simulink model "Simulations_section74"  (R2023a)
settings: Solver=ode15s  StartTime=0.0  StopTime=time_end  FixedStep=Ts  MaxStep=1e-3  RelTol=1e-3
values from neighbouring files (symbols this model uses):
  Akmax = CorrM.a    [Section74.m]
  Akmin = Corrm.a    [Section74.m]
  Bkmax = CorrM.b    [Section74.m]
  Bkmin = Corrm.b    [Section74.m]
  Ckmax = CorrM.c    [Section74.m]
  Ckmin = Corrm.c    [Section74.m]
  rhomax = 0.99    [Section74.m]
  rhomin = 0.01    [Section74.m]
  scenario = input('Which scenario would you like to run: 1 or 2 ? Answer = ')    [Section74.m]
undefined symbols (not defined in the file or in its folder): sigbuilder_block
libraries: cstblocks x6
settings Model: ExtModeTrigDuration=100000  Creator=senameo  LastModifiedBy=senameo
settings DataIOCC: SaveFormat=Array  SignalLoggingSaveFormat=ModelDataLogs  ReturnWorkspaceOutputs=off
settings OptimizationCC: BlockReduction=off  BooleanDataType=off  InitFltsAndDblsToZero=on  LifeSpan=inf
settings DebuggingCC: SaveWithParameterizedLinksMsg=none  UnderspecifiedInitializationDetection=Classic  MergeDetectMultiDrivingBlocksExec=none  SignalResolutionControl=TryResolveAllWithWarning  MultiTaskDSMMsg=warning  MultiTaskCondExecSysMsg=none  FcnCallInpInsideContextMsg=warning  UnconnectedInputMsg=warning  UnconnectedOutputMsg=warning  UnconnectedLineMsg=warning  SFUnexpectedBacktrackingDiag=warning  SFNoUnconditionalDefaultTransitionDiag=warning  SFExecutionAtInitializationDiag=none  ArithmeticOperatorsInVariantConditions=warning
settings HardwareCC: ProdBitPerPointer=32  ProdBitPerSizeT=32  ProdBitPerPtrDiffT=32  ProdLargestAtomicFloat=None  ProdIntDivRoundTo=Undefined  ProdEndianess=Unspecified  ProdWordSize=32  ProdHWDeviceType=32-bit Generic  TargetUnknown=on
settings ModelReferenceCC: EnableRefExpFcnMdlSchedulingChecks=on  PropagateSignalLabelsOutOfModel=off
settings RTWCC: SystemTargetFile=win_watc.tlc  TemplateMakefile=win_watc.tmf  DLArmComputeVersion=19.05
settings CodeAppCC: StateflowObjectComments=on
settings STFCustomTargetCC: TargetFcnLib=ansi_tfl_tmw.mat  TargetLangStandard=C89/C90 (ANSI)  ModelReferenceCompliant=off  ConcurrentExecutionCompliant=off  MATLABClassNameForMDSCustomization=Simulink.SoftwareTarget.TargetSpecificTriggerConfigurationBase  UseToolchainInfoCompliant=off  SystemTargetFile=win_watc.tlc
settings ConfigComp: CovMetricSettings=dw  CovSaveCumulativeToWorkspaceVar=on  CovSaveSingleToWorkspaceVar=on

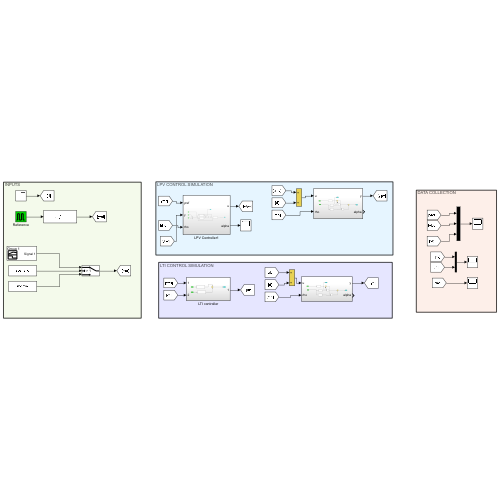
[thumbnail: Simulink's stored preview of the top-level diagram]
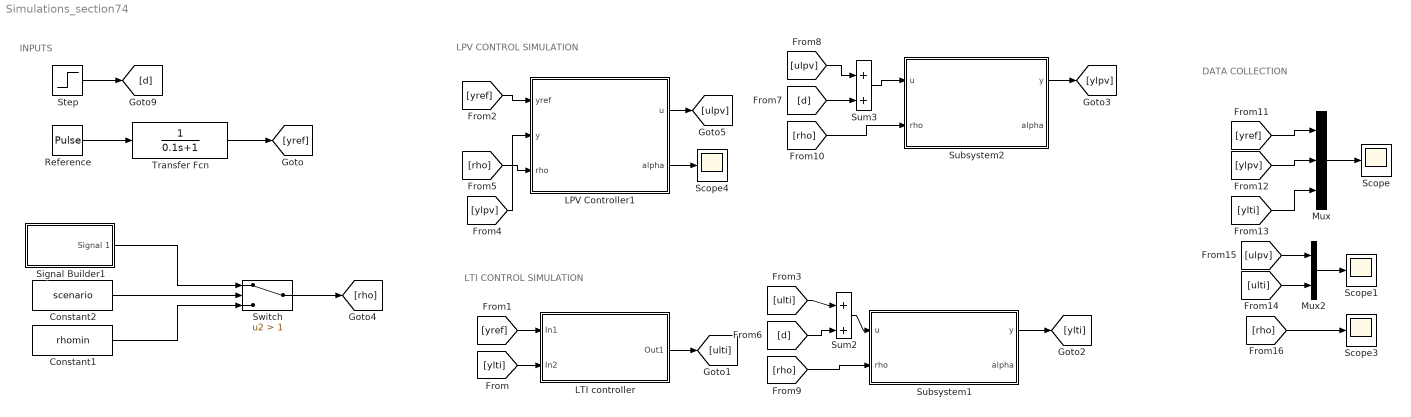
== system Simulations_section74 ==
  note: DATA COLLECTION
  note: LPV CONTROL SIMULATION
  note: LTI CONTROL SIMULATION
  note: INPUTS
  Constant1 : Constant  Value=rhomin
  Constant2 : Constant  Value=scenario
  LPV Controller1 : Subsystem
  LTI controller : Subsystem
  Mux : Mux  Inputs=3
  Mux2 : Mux  Inputs=2
  Reference : DiscretePulseGenerator  PulseType=Time based  Period=30  PulseWidth=50  PhaseDelay=1
  Scope{,1,3..4} (4 alike) : Scope
  Signal Builder1 : Subsystem  Tag=STV Subsys  LoadFcn=sigbuilder_block('load');  StartFcn=sigbuilder_block('start');  StopFcn=sigbuilder_block('stop');  ClipboardFcn=sigbuilder_block('clipboard');  mask(Sigbuilder block){tuvar=[0:10]}
      mask help: Simulink:masks:SigbuilderBlock_MD
      mask init:
      | if ~strcmp(get_param(bdroot(gcbh),'SimulationStatus'),'stopped') tuvar = sigbuilder_block('maskInit'); end
      settings: CopyFcn=sigbuilder_block('copy');  DeleteFcn=sigbuilder_block('delete');  ModelCloseFcn=sigbuilder_block('modelClose');  PreSaveFcn=sigbuilder_block('preSave');  PauseFcn=sigbuilder_block('pause');  ContinueFcn=sigbuilder_block('continue');  NameChangeFcn=sigbuilder_block('namechange');  OpenFcn=sigbuilder_block('open',[597 9 550.2 191.1 ]);  CloseFcn=sigbuilder_block('close');
      mask Display: plot(0, 0, 100, 100,[2, 2, 32, 32, 2], [68, 8, 8, 68, 68],[32, 2], [38, 38], [32, 19, 2],[53, 60, 44], [32, 17, 17, 2],[16, 16, 31, 31]);txt = getActiveGroup(gcbh);text(2, 100, txt,'verticalAlignment', 'top');
  Step : Step  Time=20  After=0.1  SampleTime=0
  Subsystem1 : Subsystem
  Subsystem2 : Subsystem
  Sum2 : Sum  Inputs=+|+  InputSameDT=on  SaturateOnIntegerOverflow=on  OutDataTypeStr=Inherit: Same as first input
  Sum3 : Sum  Inputs=+|+  InputSameDT=on  SaturateOnIntegerOverflow=on  OutDataTypeStr=Inherit: Same as first input
  Switch : Switch  Criteria=u2 > Threshold  Threshold=1  SaturateOnIntegerOverflow=off  InputSameDT=off
  Transfer Fcn : TransferFcn  Denominator=[0.1 1]
  wires:
  Sum2/1 -> Subsystem1/1(u)
  Mux2/1 -> Scope1/1
  Transfer Fcn/1 -> [yref]
  Reference/1 -> Transfer Fcn/1
  Mux/1 -> Scope/1
  [yref] -> LTI controller/1(In1)
  [ylti] -> LTI controller/2(In2)
  LTI controller/1(Out1) -> [ulti]
  [ulti] -> Sum2/1
  [d] -> Sum2/2
  [rho] -> Subsystem1/2(rho)
  [yref] -> Mux/1
  Subsystem1/1(y) -> [ylti]
  [ylpv] -> Mux/2
  [ulti] -> Mux2/2
  [ulpv] -> Mux2/1
  Constant2/1 -> Switch/2
  Switch/1 -> [rho]
  Step/1 -> [d]
  Constant1/1 -> Switch/3
  Signal Builder1/1(Signal 1) -> Switch/1
  [ylti] -> Mux/3
  Subsystem2/1(y) -> [ylpv]
  [ulpv] -> Sum3/1
  [rho] -> LPV Controller1/3(rho)
  LPV Controller1/1(u) -> [ulpv]
  [d] -> Sum3/2
  [yref] -> LPV Controller1/1(yref)
  [rho] -> Subsystem2/2(rho)
  Sum3/1 -> Subsystem2/1(u)
  [ylpv] -> LPV Controller1/2(y)
  LPV Controller1/2(alpha) -> Scope4/1
  [rho] -> Scope3/1

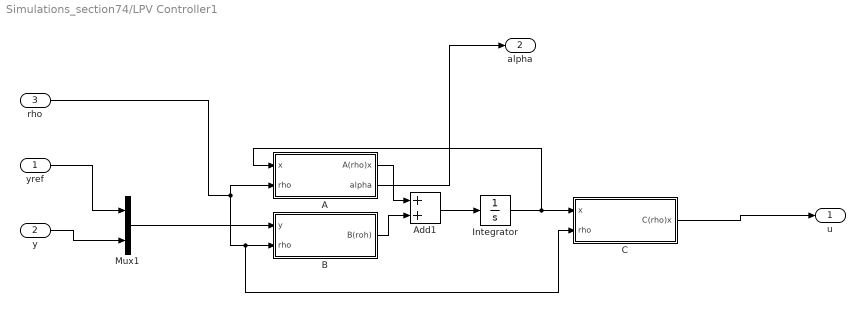
== system Simulations_section74/LPV Controller1 ==
  yref : Inport
  y : Inport  Port=2
  rho : Inport  Port=3
  A : Subsystem
  Add1 : Sum
  B : Subsystem
  C : Subsystem
  Integrator : Integrator
  Mux1 : Mux  Inputs=2
  u : Outport  VectorParamsAs1DForOutWhenUnconnected=off
  alpha : Outport  Port=2  VectorParamsAs1DForOutWhenUnconnected=off
  wires:
  Mux1/1 -> B/1(y)
  yref/1 -> Mux1/1
  C/1(C(rho)x) -> u/1
  rho/1 -> C/2(rho), B/2(rho), A/2(rho)
  A/1(A(rho)x) -> Add1/1
  B/1(B(roh)) -> Add1/2
  Add1/1 -> Integrator/1
  Integrator/1 -> A/1(x), C/1(x)
  A/2(alpha) -> alpha/1
  y/1 -> Mux1/2

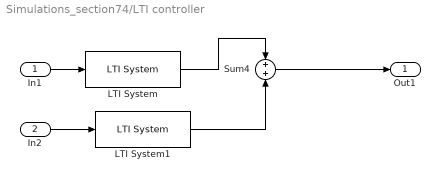
== system Simulations_section74/LTI controller ==
  In1 : Inport
  In2 : Inport  Port=2
  LTI System : cstblocks/LTI System  sys=Kr  IC=[]
  LTI System1 : cstblocks/LTI System  sys=Ky  IC=[]
  Sum4 : Sum  InputSameDT=on  SaturateOnIntegerOverflow=on  OutDataTypeStr=Inherit: Same as first input
  Out1 : Outport
  wires:
  In2/1 -> LTI System1/1
  LTI System/1 -> Sum4/1
  In1/1 -> LTI System/1
  LTI System1/1 -> Sum4/2
  Sum4/1 -> Out1/1

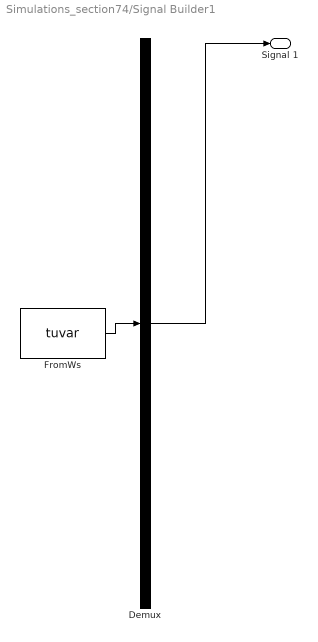
== system Simulations_section74/Signal Builder1 ==
  Demux : Demux  Tag=STV Demux  Outputs=1
      settings: DisplayOption=none
  FromWs : FromWorkspace  Tag=STV FromWs  VariableName=tuvar
      SigBuilderData=|
      | common.afterFinalStr = 'Extrapolate'
      | common.sampleTime = 0
      | dataSet.timeRange = [0 90]
      | dataSet.name = 'Group 1'
      | sbobj.Groups.Name = 'Group 1'
      | sbobj.Groups.Signals.Name = 'Signal 1'
      | sbobj.Groups.Signals.XData = [0 40 40 50 80 90]
      | sbobj.Groups.Signals.YData = [0 0 0.5 0.5 0.9 0.9]
      | sbobj.Groups.TimeRange = [0 90]
  Signal 1 : Outport  Tag=STV Outport
  wires:
  Demux/1 -> Signal 1/1
  FromWs/1 -> Demux/1

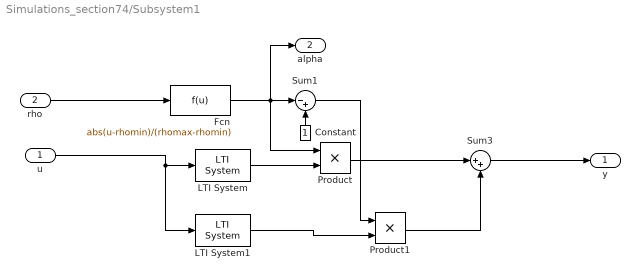
== system Simulations_section74/Subsystem1 ==
  u : Inport
  rho : Inport  Port=2
  Constant : Constant
  Fcn : Fcn  Expr=abs(u-rhomin)/(rhomax-rhomin)
  LTI System : cstblocks/LTI System  sys=model_100  IC=[]
  LTI System1 : cstblocks/LTI System  sys=model_0  IC=[]
  Product : Product  RndMeth=Zero
  Product1 : Product  RndMeth=Zero
  Sum1 : Sum  Inputs=|-+  InputSameDT=on  SaturateOnIntegerOverflow=on  OutDataTypeStr=Inherit: Same as first input
  Sum3 : Sum  Inputs=|++  InputSameDT=on  SaturateOnIntegerOverflow=on  OutDataTypeStr=Inherit: Same as first input
  y : Outport
  alpha : Outport  Port=2
  wires:
  LTI System1/1 -> Product1/2
  LTI System/1 -> Product/2
  rho/1 -> Fcn/1
  Constant/1 -> Sum1/2
  Sum3/1 -> y/1
  Product1/1 -> Sum3/2
  Fcn/1 -> Product/1, alpha/1, Sum1/1
  Product/1 -> Sum3/1
  Sum1/1 -> Product1/1
  u/1 -> LTI System1/1, LTI System/1

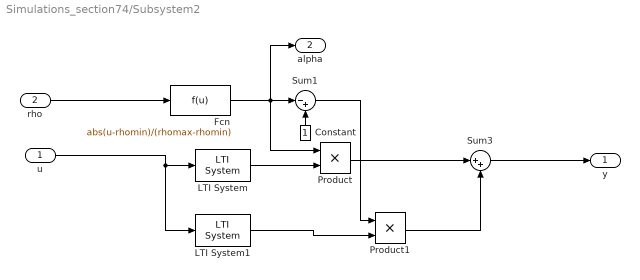
== system Simulations_section74/Subsystem2 ==
  u : Inport
  rho : Inport  Port=2
  Constant : Constant
  Fcn : Fcn  Expr=abs(u-rhomin)/(rhomax-rhomin)
  LTI System : cstblocks/LTI System  sys=model_100  IC=[]
  LTI System1 : cstblocks/LTI System  sys=model_0  IC=[]
  Product : Product  RndMeth=Zero
  Product1 : Product  RndMeth=Zero
  Sum1 : Sum  Inputs=|-+  InputSameDT=on  SaturateOnIntegerOverflow=on  OutDataTypeStr=Inherit: Same as first input
  Sum3 : Sum  Inputs=|++  InputSameDT=on  SaturateOnIntegerOverflow=on  OutDataTypeStr=Inherit: Same as first input
  y : Outport
  alpha : Outport  Port=2
  wires:
  LTI System1/1 -> Product1/2
  LTI System/1 -> Product/2
  rho/1 -> Fcn/1
  Constant/1 -> Sum1/2
  Sum3/1 -> y/1
  Product1/1 -> Sum3/2
  Fcn/1 -> Product/1, alpha/1, Sum1/1
  Product/1 -> Sum3/1
  Sum1/1 -> Product1/1
  u/1 -> LTI System1/1, LTI System/1

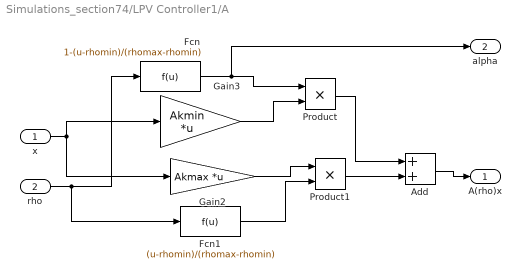
== system Simulations_section74/LPV Controller1/A ==
  x : Inport
  rho : Inport  Port=2
  Add : Sum
  Fcn : Fcn  Expr=1-(u-rhomin)/(rhomax-rhomin)
  Fcn1 : Fcn  Expr=(u-rhomin)/(rhomax-rhomin)
  Gain2 : Gain  Gain=Akmax  Multiplication=Matrix(K*u)
  Gain3 : Gain  Gain=Akmin  Multiplication=Matrix(K*u)
  Product : Product
  Product1 : Product
  A(rho)x : Outport  VectorParamsAs1DForOutWhenUnconnected=off
  alpha : Outport  Port=2  VectorParamsAs1DForOutWhenUnconnected=off
  wires:
  Gain2/1 -> Product1/1
  Gain3/1 -> Product/2
  Fcn1/1 -> Product1/2
  Fcn/1 -> alpha/1, Product/1
  Add/1 -> A(rho)x/1
  Product1/1 -> Add/2
  Product/1 -> Add/1
  rho/1 -> Fcn1/1, Fcn/1
  x/1 -> Gain2/1, Gain3/1

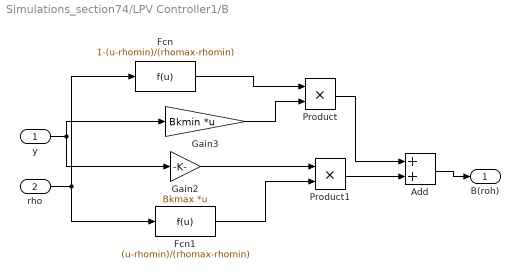
== system Simulations_section74/LPV Controller1/B ==
  y : Inport
  rho : Inport  Port=2
  Add : Sum
  Fcn : Fcn  Expr=1-(u-rhomin)/(rhomax-rhomin)
  Fcn1 : Fcn  Expr=(u-rhomin)/(rhomax-rhomin)
  Gain2 : Gain  Gain=Bkmax  Multiplication=Matrix(K*u)
  Gain3 : Gain  Gain=Bkmin  Multiplication=Matrix(K*u)
  Product : Product
  Product1 : Product
  B(roh) : Outport  VectorParamsAs1DForOutWhenUnconnected=off
  wires:
  Gain2/1 -> Product1/1
  Gain3/1 -> Product/2
  Fcn1/1 -> Product1/2
  Fcn/1 -> Product/1
  Add/1 -> B(roh)/1
  Product1/1 -> Add/2
  Product/1 -> Add/1
  rho/1 -> Fcn1/1, Fcn/1
  y/1 -> Gain2/1, Gain3/1

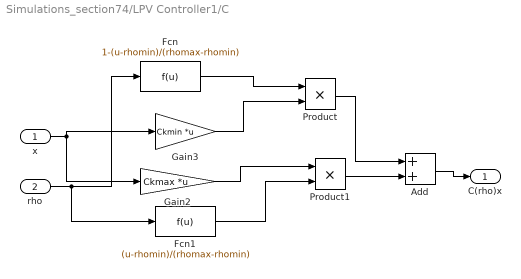
== system Simulations_section74/LPV Controller1/C ==
  x : Inport
  rho : Inport  Port=2
  Add : Sum
  Fcn : Fcn  Expr=1-(u-rhomin)/(rhomax-rhomin)
  Fcn1 : Fcn  Expr=(u-rhomin)/(rhomax-rhomin)
  Gain2 : Gain  Gain=Ckmax  Multiplication=Matrix(K*u)
  Gain3 : Gain  Gain=Ckmin  Multiplication=Matrix(K*u)
  Product : Product
  Product1 : Product
  C(rho)x : Outport  VectorParamsAs1DForOutWhenUnconnected=off
  wires:
  Gain2/1 -> Product1/1
  Gain3/1 -> Product/2
  Fcn1/1 -> Product1/2
  Fcn/1 -> Product/1
  Add/1 -> C(rho)x/1
  Product1/1 -> Add/2
  Product/1 -> Add/1
  rho/1 -> Fcn1/1, Fcn/1
  x/1 -> Gain2/1, Gain3/1
